simulink model "HConstfolding_export"  (Simulink 7.9)
settings: Solver=ode45  StartTime=0.0  StopTime=10.0  RelTol=1e-3
settings Model: Creator=boakes  LastModifiedBy=boakes

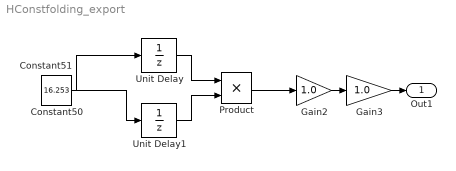
== system HConstfolding_export ==
  Constant50 : Constant  Value=36.6
  Constant51 : Constant  Value=16.253
  Gain2 : Gain  Gain=1.0
  Gain3 : Gain  Gain=1.0
  Product : Product  RndMeth=Zero
  Unit Delay : UnitDelay  X0=0.0  SampleTime=-1.0
  Unit Delay1 : UnitDelay  X0=0.0  SampleTime=-1.0
  Out1 : Outport
  wires:
  Gain2/1 -> Gain3/1
  Product/1 -> Gain2/1
  Gain3/1 -> Out1/1
  Constant50/1 -> Unit Delay1/1
  Unit Delay1/1 -> Product/2
  Constant51/1 -> Unit Delay/1
  Unit Delay/1 -> Product/1
